simulink model "sim_doubint"  (Simulink 6.2)
settings: Solver=ode45  SolverMode=SingleTasking  StartTime=0.0  StopTime=Tmax  MaxStep=0.01  RelTol=1e-3
undefined symbols (not defined in the file or in its folder): dK, nK, T
settings Model: LastModifiedBy=Administrator
settings DataIOCC: SignalLoggingName=sigsOut
settings OptimizationCC: BooleanDataType=off  InlineInvariantSignals=on
settings HardwareCC: TargetUnknown=on

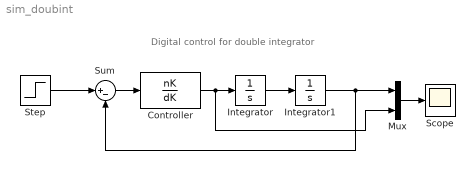
== system sim_doubint ==
  note: Digital control for double integrator
  Controller : DiscreteTransferFcn  Numerator=nK  Denominator=dK  SampleTime=T
  Integrator : Integrator
  Integrator1 : Integrator
  Mux : Mux  Inputs=2
  Scope : Scope
      settings: TimeRange=3  YMin=-0.08  YMax=0.09999999999999999  SaveName=out  DataFormat=Array
  Step : Step  Time=0  SampleTime=0
  Sum : Sum  Inputs=|+-
  wires:
  Step/1 -> Sum/1
  Sum/1 -> Controller/1
  Controller/1 -> Integrator/1, Mux/2
  Integrator/1 -> Integrator1/1
  Integrator1/1 -> Sum/2, Mux/1
  Mux/1 -> Scope/1
